simulink model "DISCON_NREL5MW_WaveFF"  (R2022a)
settings: Solver=FixedStepDiscrete  StartTime=0.0  StopTime=inf  FixedStep=Control.TimeStep  RelTol=1e-3
values from neighbouring files (symbols this model uses):
  Gd_Fwave = c2d(Sys{OperatingPoint}('omega_r','F_{hydro}'),Control.TimeStep,'tustin')    [ControlParams_NREL5MW.m]
  Gd_Mwave = c2d(Sys{OperatingPoint}('omega_r','M_{hydro}'),Control.TimeStep,'tustin')    [ControlParams_NREL5MW.m]
  InvGp = inv(Gp)    [ControlParams_NREL5MW.m]
  Kff_gain = 0.3    [InitCompDISCON.m]
undefined symbols (not defined in the file or in its folder): Control
settings Model: Creator=evansolingen  LastModifiedBy=Amr Hegazy
settings SolverCC: AlgebraicLoopSolver=TrustRegion
settings DataIOCC: LimitDataPoints=on  SaveFormat=Array  SignalLoggingSaveFormat=ModelDataLogs  SaveOutput=off  SignalLogging=off  SaveTime=off  ReturnWorkspaceOutputs=off
settings OptimizationCC: ExpressionDepthLimit=2147483647  LifeSpan=inf
settings DebuggingCC: UnderspecifiedInitializationDetection=Classic  MergeDetectMultiDrivingBlocksExec=none  SolverPrmCheckMsg=warning  MultiTaskDSMMsg=warning  MultiTaskCondExecSysMsg=none  FcnCallInpInsideContextMsg=warning  UnconnectedInputMsg=warning  UnconnectedOutputMsg=warning  UnconnectedLineMsg=warning  AllowSymbolicDim=off  StateNameClashWarn=warning  SFUnexpectedBacktrackingDiag=warning  SFNoUnconditionalDefaultTransitionDiag=warning  SFExecutionAtInitializationDiag=none  SFMachineParentedDataDiag=warning  ArithmeticOperatorsInVariantConditions=warning
settings HardwareCC: ProdBitPerPointer=32  ProdBitPerSizeT=32  ProdBitPerPtrDiffT=32  ProdLargestAtomicFloat=None  ProdIntDivRoundTo=Undefined  ProdEndianess=Unspecified  ProdWordSize=32  ProdHWDeviceType=32-bit Generic
settings ModelReferenceCC: UpdateModelReferenceTargets=Force  PropagateSignalLabelsOutOfModel=off
settings SFSimCC: SimUseLocalCustomCode=off  SimParseCustomCode=off  CustomCodeUndefinedFunction=UseInterfaceOnly
settings RTWCC: Description=DISCON DLL Target (for use with GH BLADED)  SystemTargetFile=discon.tlc  TemplateMakefile=discon_vc.tmf  RTWUseLocalCustomCode=off
settings CodeAppCC: StateflowObjectComments=on
settings GRTTargetCC: TargetLangStandard=C89/C90 (ANSI)  CombineOutputUpdateFcns=off  GRTInterface=on  UseToolchainInfoCompliant=off  ExtModeMexFile=noextcomm
settings ConfigComp: CovMetricSettings=dw  CovSaveCumulativeToWorkspaceVar=on  CovSaveSingleToWorkspaceVar=on  CovExternalEMLEnable=off

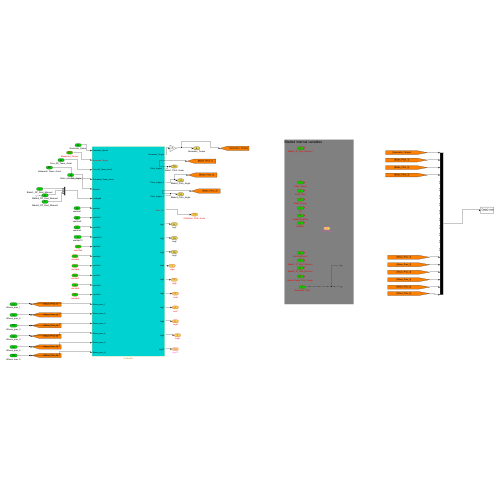
[thumbnail: Simulink's stored preview of the top-level diagram]
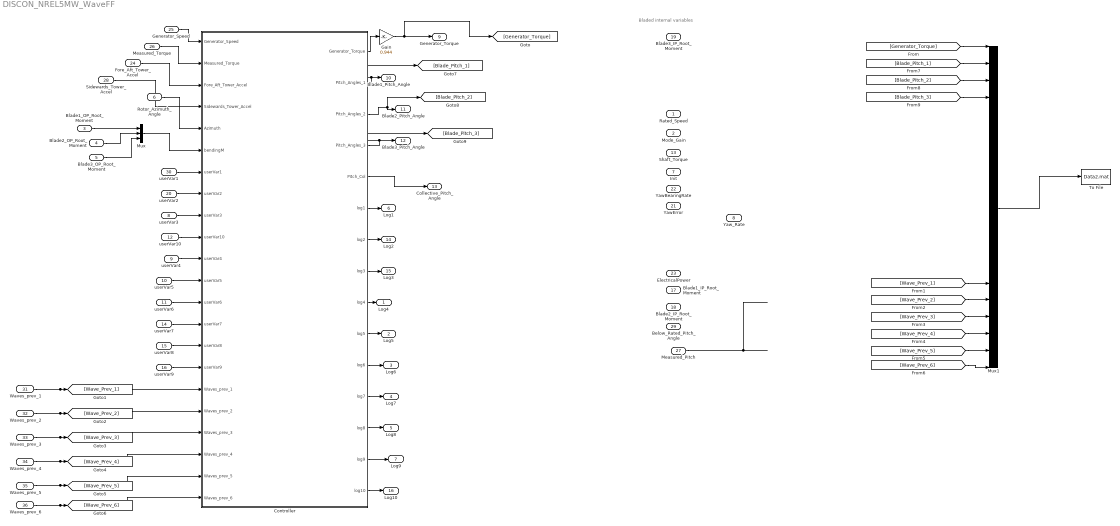
== system DISCON_NREL5MW_WaveFF ==
  note: Bladed internal variables
  Rated_Speed : Inport  PortDimensions=1
  Mode_Gain : Inport  Port=2  PortDimensions=1
  Blade1_OP_Root_Moment : Inport  Port=3  PortDimensions=1
  Blade2_OP_Root_Moment : Inport  Port=4  PortDimensions=1
  Blade3_OP_Root_Moment : Inport  Port=5  PortDimensions=1
  Rotor_Azimuth_Angle : Inport  Port=6  PortDimensions=1
  Init : Inport  Port=7  PortDimensions=1
  userVar3 : Inport  Port=8  PortDimensions=1
  userVar4 : Inport  Port=9  PortDimensions=1
  userVar5 : Inport  Port=10  PortDimensions=1
  userVar6 : Inport  Port=11  PortDimensions=1
  userVar10 : Inport  Port=12  PortDimensions=1
  Shaft_Torque : Inport  Port=13  PortDimensions=1
  userVar7 : Inport  Port=14  PortDimensions=1
  userVar8 : Inport  Port=15  PortDimensions=1
  userVar9 : Inport  Port=16  PortDimensions=1
  Blade1_IP_Root_Moment : Inport  Port=17  PortDimensions=1
  Blade2_IP_Root_Moment : Inport  Port=18  PortDimensions=1
  Blade3_IP_Root_Moment : Inport  Port=19  PortDimensions=1
  userVar2 : Inport  Port=20  PortDimensions=1
  YawError : Inport  Port=21  PortDimensions=1
  YawBearingRate : Inport  Port=22  PortDimensions=1
  ElectricalPower : Inport  Port=23  PortDimensions=1
  Fore_Aft_Tower_Accel : Inport  Port=24  PortDimensions=1
  Generator_Speed : Inport  Port=25  PortDimensions=1
  Measured_Torque : Inport  Port=26  PortDimensions=1
  Measured_Pitch : Inport  Port=27  PortDimensions=1
  Sidewards_Tower_Accel : Inport  Port=28  PortDimensions=1
  Below_Rated_Pitch_Angle : Inport  Port=29  PortDimensions=1
  userVar1 : Inport  Port=30  PortDimensions=1
  Waves_prev_1 : Inport  Port=31  PortDimensions=1
  Waves_prev_2 : Inport  Port=32  PortDimensions=1
  Waves_prev_3 : Inport  Port=33  PortDimensions=1
  Waves_prev_4 : Inport  Port=34  PortDimensions=1
  Waves_prev_5 : Inport  Port=35  PortDimensions=1
  Waves_prev_6 : Inport  Port=36  PortDimensions=1
  Controller : Subsystem
  Gain : Gain  Gain=0.944
  Mux : Mux  Inputs=3
  Mux1 : Mux  Inputs=20
  To File : ToFile  Filename=Data2.mat
  Log4 : Outport  PortDimensions=1  VectorParamsAs1DForOutWhenUnconnected=off
  Log5 : Outport  Port=2  PortDimensions=1  VectorParamsAs1DForOutWhenUnconnected=off
  Log6 : Outport  Port=3  PortDimensions=1  VectorParamsAs1DForOutWhenUnconnected=off
  Log7 : Outport  Port=4  PortDimensions=1  VectorParamsAs1DForOutWhenUnconnected=off
  Log8 : Outport  Port=5  PortDimensions=1  VectorParamsAs1DForOutWhenUnconnected=off
  Log1 : Outport  Port=6  PortDimensions=1  VectorParamsAs1DForOutWhenUnconnected=off
  Log9 : Outport  Port=7  PortDimensions=1  VectorParamsAs1DForOutWhenUnconnected=off
  Yaw_Rate : Outport  Port=8  PortDimensions=1  VectorParamsAs1DForOutWhenUnconnected=off
  Generator_Torque : Outport  Port=9  PortDimensions=1  VectorParamsAs1DForOutWhenUnconnected=off
  Blade1_Pitch_Angle : Outport  Port=10  PortDimensions=1  VectorParamsAs1DForOutWhenUnconnected=off
  Blade2_Pitch_Angle : Outport  Port=11  PortDimensions=1  VectorParamsAs1DForOutWhenUnconnected=off
  Blade3_Pitch_Angle : Outport  Port=12  PortDimensions=1  VectorParamsAs1DForOutWhenUnconnected=off
  Collective_Pitch_Angle : Outport  Port=13  PortDimensions=1  VectorParamsAs1DForOutWhenUnconnected=off
  Log2 : Outport  Port=14  PortDimensions=1  VectorParamsAs1DForOutWhenUnconnected=off
  Log3 : Outport  Port=15  PortDimensions=1  VectorParamsAs1DForOutWhenUnconnected=off
  Log10 : Outport  Port=16  PortDimensions=1  VectorParamsAs1DForOutWhenUnconnected=off
  wires:
  Fore_Aft_Tower_Accel/1 -> Controller/3(Fore_Aft_Tower_Accel)
  Measured_Pitch/1 -> ?
  ? -> ?
  Generator_Speed/1 -> Controller/1(Generator_Speed)
  Controller/1(Generator_Torque) -> Gain/1
  userVar3/1 -> Controller/9(userVar3)
  Gain/1 -> Generator_Torque/1, [Generator_Torque]
  Measured_Torque/1 -> Controller/2(Measured_Torque)
  Sidewards_Tower_Accel/1 -> Controller/4(Sidewards_Tower_Accel)
  Rotor_Azimuth_Angle/1 -> Controller/5(Azimuth)
  Blade1_OP_Root_Moment/1 -> Mux/1
  Blade2_OP_Root_Moment/1 -> Mux/2
  Blade3_OP_Root_Moment/1 -> Mux/3
  Mux/1 -> Controller/6(bendingM)
  Controller/2(Pitch_Angles_1) -> Blade1_Pitch_Angle/1, [Blade_Pitch_1]
  Controller/3(Pitch_Angles_2) -> [Blade_Pitch_2], Blade2_Pitch_Angle/1
  Controller/4(Pitch_Angles_3) -> Blade3_Pitch_Angle/1, [Blade_Pitch_3]
  Controller/5(Pitch_Col) -> Collective_Pitch_Angle/1
  userVar1/1 -> Controller/7(userVar1)
  userVar2/1 -> Controller/8(userVar2)
  userVar10/1 -> Controller/10(userVar10)
  Mux1/1 -> To File/1
  [Generator_Torque] -> Mux1/1
  Waves_prev_1/1 -> Controller/17(Waves_prev_1), [Wave_Prev_1]
  Waves_prev_2/1 -> Controller/18(Waves_prev_2), [Wave_Prev_2]
  Waves_prev_3/1 -> Controller/19(Waves_prev_3), [Wave_Prev_3]
  Waves_prev_4/1 -> Controller/20(Waves_prev_4), [Wave_Prev_4]
  Waves_prev_5/1 -> Controller/21(Waves_prev_5), [Wave_Prev_5]
  Waves_prev_6/1 -> Controller/22(Waves_prev_6), [Wave_Prev_6]
  [Wave_Prev_6] -> Mux1/20
  [Wave_Prev_5] -> Mux1/19
  [Wave_Prev_4] -> Mux1/18
  [Wave_Prev_3] -> Mux1/17
  [Wave_Prev_2] -> Mux1/16
  [Wave_Prev_1] -> Mux1/15
  [Blade_Pitch_1] -> Mux1/2
  [Blade_Pitch_2] -> Mux1/3
  [Blade_Pitch_3] -> Mux1/4
  userVar4/1 -> Controller/11(userVar4)
  userVar5/1 -> Controller/12(userVar5)
  userVar6/1 -> Controller/13(userVar6)
  userVar7/1 -> Controller/14(userVar7)
  userVar8/1 -> Controller/15(userVar8)
  userVar9/1 -> Controller/16(userVar9)
  Controller/6(log1) -> Log1/1
  Controller/7(log2) -> Log2/1
  Controller/8(log3) -> Log3/1
  Controller/10(log5) -> Log5/1
  Controller/12(log7) -> Log7/1
  Controller/13(log8) -> Log8/1
  Controller/9(log4) -> Log4/1
  Controller/15(log10) -> Log10/1
  Controller/11(log6) -> Log6/1
  Controller/14(log9) -> Log9/1

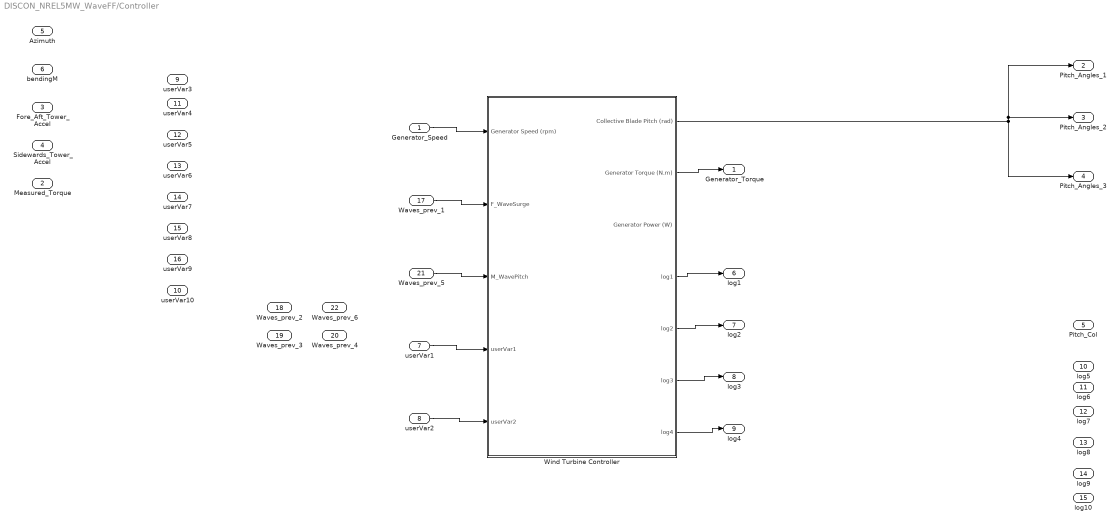
== system DISCON_NREL5MW_WaveFF/Controller ==
  Generator_Speed : Inport
  Measured_Torque : Inport  Port=2
  Fore_Aft_Tower_Accel : Inport  Port=3
  Sidewards_Tower_Accel : Inport  Port=4  PortDimensions=1
  Azimuth : Inport  Port=5  PortDimensions=1
  bendingM : Inport  Port=6
  userVar1 : Inport  Port=7  PortDimensions=1
  userVar2 : Inport  Port=8  PortDimensions=1
  userVar3 : Inport  Port=9  PortDimensions=1
  userVar10 : Inport  Port=10  PortDimensions=1
  userVar4 : Inport  Port=11  PortDimensions=1
  userVar5 : Inport  Port=12  PortDimensions=1
  userVar6 : Inport  Port=13  PortDimensions=1
  userVar7 : Inport  Port=14  PortDimensions=1
  userVar8 : Inport  Port=15  PortDimensions=1
  userVar9 : Inport  Port=16  PortDimensions=1
  Waves_prev_1 : Inport  Port=17  PortDimensions=1
  Waves_prev_2 : Inport  Port=18  PortDimensions=1
  Waves_prev_3 : Inport  Port=19  PortDimensions=1
  Waves_prev_4 : Inport  Port=20  PortDimensions=1
  Waves_prev_5 : Inport  Port=21  PortDimensions=1
  Waves_prev_6 : Inport  Port=22  PortDimensions=1
  Wind Turbine Controller : Subsystem
  Generator_Torque : Outport  VectorParamsAs1DForOutWhenUnconnected=off
  Pitch_Angles_1 : Outport  Port=2  PortDimensions=1  VectorParamsAs1DForOutWhenUnconnected=off
  Pitch_Angles_2 : Outport  Port=3  PortDimensions=1  VectorParamsAs1DForOutWhenUnconnected=off
  Pitch_Angles_3 : Outport  Port=4  PortDimensions=1  VectorParamsAs1DForOutWhenUnconnected=off
  Pitch_Col : Outport  Port=5  PortDimensions=1  VectorParamsAs1DForOutWhenUnconnected=off
  log1 : Outport  Port=6  PortDimensions=1  VectorParamsAs1DForOutWhenUnconnected=off
  log2 : Outport  Port=7  PortDimensions=1  VectorParamsAs1DForOutWhenUnconnected=off
  log3 : Outport  Port=8  PortDimensions=1  VectorParamsAs1DForOutWhenUnconnected=off
  log4 : Outport  Port=9  PortDimensions=1  VectorParamsAs1DForOutWhenUnconnected=off
  log5 : Outport  Port=10  PortDimensions=1  VectorParamsAs1DForOutWhenUnconnected=off
  log6 : Outport  Port=11  PortDimensions=1  VectorParamsAs1DForOutWhenUnconnected=off
  log7 : Outport  Port=12  PortDimensions=1  VectorParamsAs1DForOutWhenUnconnected=off
  log8 : Outport  Port=13  PortDimensions=1  VectorParamsAs1DForOutWhenUnconnected=off
  log9 : Outport  Port=14  PortDimensions=1  VectorParamsAs1DForOutWhenUnconnected=off
  log10 : Outport  Port=15  PortDimensions=1  VectorParamsAs1DForOutWhenUnconnected=off
  wires:
  Wind Turbine Controller/2(Generator Torque (N.m)) -> Generator_Torque/1
  Waves_prev_5/1 -> Wind Turbine Controller/3(M_WavePitch)
  Waves_prev_1/1 -> Wind Turbine Controller/2(F_WaveSurge)
  Generator_Speed/1 -> Wind Turbine Controller/1(Generator Speed (rpm))
  userVar1/1 -> Wind Turbine Controller/4(userVar1)
  userVar2/1 -> Wind Turbine Controller/5(userVar2)
  Wind Turbine Controller/4(log1) -> log1/1
  Wind Turbine Controller/5(log2) -> log2/1
  Wind Turbine Controller/6(log3) -> log3/1
  Wind Turbine Controller/7(log4) -> log4/1
  Wind Turbine Controller/1(" Collective Blade Pitch (rad)") -> Pitch_Angles_2/1, Pitch_Angles_1/1, Pitch_Angles_3/1

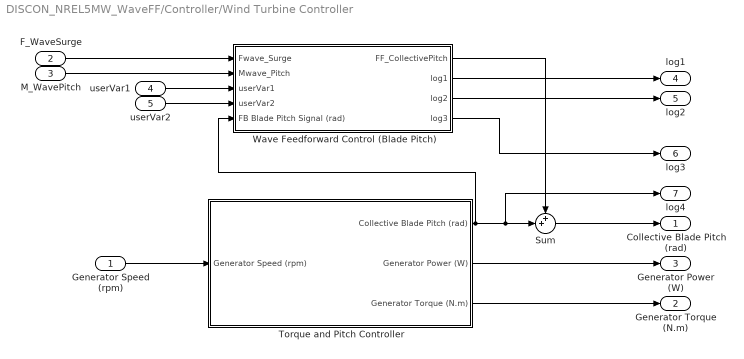
== system DISCON_NREL5MW_WaveFF/Controller/Wind Turbine Controller ==
  Generator Speed (rpm) : Inport
  F_WaveSurge : Inport  Port=2
  M_WavePitch : Inport  Port=3
  userVar1 : Inport  Port=4  PortDimensions=1
  userVar2 : Inport  Port=5  PortDimensions=1
  Sum : Sum  Inputs=++|
  Torque and Pitch Controller : Subsystem
  Wave Feedforward Control (Blade Pitch) : Subsystem
  " Collective Blade Pitch (rad)" : Outport
  Generator Torque (N.m) : Outport  Port=2
  Generator Power (W) : Outport  Port=3
  log1 : Outport  Port=4  PortDimensions=1  VectorParamsAs1DForOutWhenUnconnected=off
  log2 : Outport  Port=5  PortDimensions=1  VectorParamsAs1DForOutWhenUnconnected=off
  log3 : Outport  Port=6  PortDimensions=1  VectorParamsAs1DForOutWhenUnconnected=off
  log4 : Outport  Port=7  PortDimensions=1  VectorParamsAs1DForOutWhenUnconnected=off
  wires:
  Generator Speed (rpm)/1 -> Torque and Pitch Controller/1(Generator Speed (rpm))
  Torque and Pitch Controller/2(Generator Power (W)) -> Generator Power (W)/1
  Torque and Pitch Controller/3(Generator Torque (N.m)) -> Generator Torque (N.m)/1
  Wave Feedforward Control (Blade Pitch)/1(FF_CollectivePitch) -> Sum/1
  Torque and Pitch Controller/1(" Collective Blade Pitch (rad)") -> Wave Feedforward Control (Blade Pitch)/5(FB Blade Pitch Signal (rad)), log4/1, Sum/2
  Sum/1 -> " Collective Blade Pitch (rad)"/1
  Wave Feedforward Control (Blade Pitch)/2(log1) -> log1/1
  Wave Feedforward Control (Blade Pitch)/3(log2) -> log2/1
  Wave Feedforward Control (Blade Pitch)/4(log3) -> log3/1
  userVar1/1 -> Wave Feedforward Control (Blade Pitch)/3(userVar1)
  userVar2/1 -> Wave Feedforward Control (Blade Pitch)/4(userVar2)
  F_WaveSurge/1 -> Wave Feedforward Control (Blade Pitch)/1(Fwave_Surge)
  M_WavePitch/1 -> Wave Feedforward Control (Blade Pitch)/2(Mwave_Pitch)

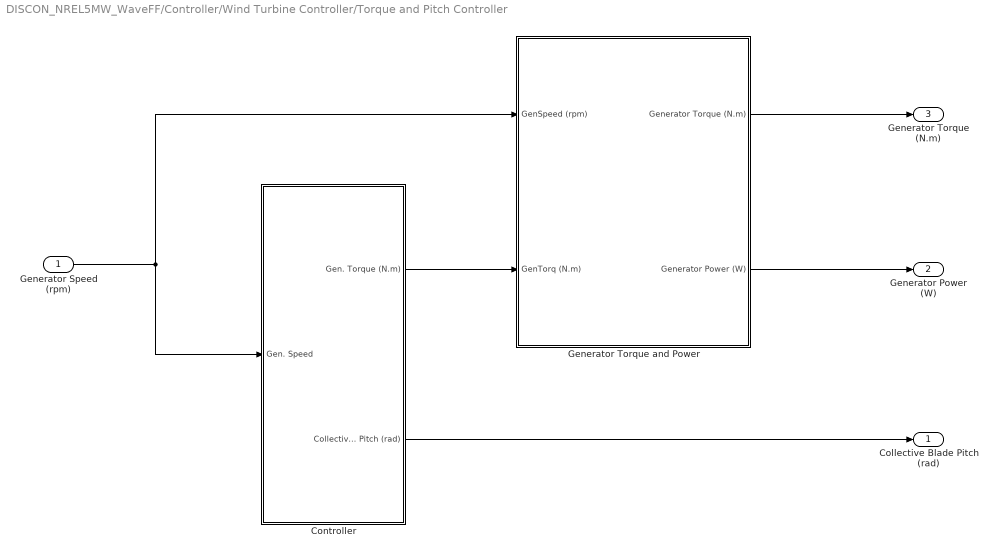
== system DISCON_NREL5MW_WaveFF/Controller/Wind Turbine Controller/Torque and Pitch Controller ==
  Generator Speed (rpm) : Inport
  Controller : Subsystem
  Generator Torque and Power : Subsystem
  " Collective Blade Pitch (rad)" : Outport
  Generator Power (W) : Outport  Port=2
  Generator Torque (N.m) : Outport  Port=3
  wires:
  Controller/1(Gen. Torque (N.m)) -> Generator Torque and Power/2(GenTorq (N.m))
  Generator Torque and Power/1(Generator Torque (N.m)) -> Generator Torque (N.m)/1
  Generator Torque and Power/2(Generator Power (W)) -> Generator Power (W)/1
  Generator Speed (rpm)/1 -> Generator Torque and Power/1(GenSpeed (rpm)), Controller/1(Gen. Speed)
  Controller/2(Collective Blade Pitch (rad)) -> " Collective Blade Pitch (rad)"/1

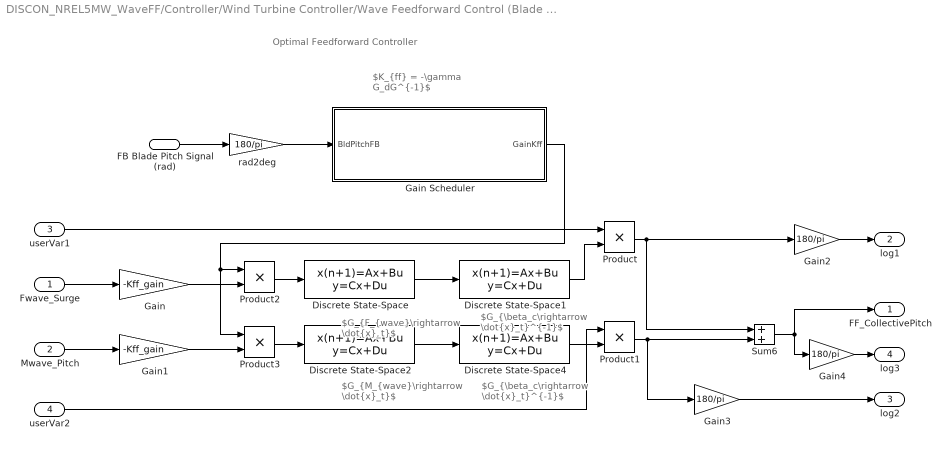
== system DISCON_NREL5MW_WaveFF/Controller/Wind Turbine Controller/Wave Feedforward Control (Blade Pitch) ==
  note: $K_{ff} = -\gamma G_dG^{-1}$
  note: Optimal Feedforward Controller
  note: $G_{F_{wave}\rightarrow \dot{x}_t}$
  note: $G_{M_{wave}\rightarrow \dot{x}_t}$
  note: $G_{\beta_c\rightarrow \dot{x}_t}^{-1}$
  note: $G_{\beta_c\rightarrow \dot{x}_t}^{-1}$
  Fwave_Surge : Inport
  Mwave_Pitch : Inport  Port=2
  userVar1 : Inport  Port=3  PortDimensions=1
  userVar2 : Inport  Port=4  PortDimensions=1
  FB Blade Pitch Signal (rad) : Inport  Port=5
  Discrete State-Space : DiscreteStateSpace  A=Gd_Fwave.A  B=Gd_Fwave.B  C=Gd_Fwave.C  D=Gd_Fwave.D  SampleTime=Control.TimeStep
  Discrete State-Space1 : DiscreteStateSpace  A=InvGp.A  B=InvGp.B  C=InvGp.C  D=InvGp.D  SampleTime=Control.TimeStep
  Discrete State-Space2 : DiscreteStateSpace  A=Gd_Mwave.A  B=Gd_Mwave.B  C=Gd_Mwave.C  D=Gd_Mwave.D  SampleTime=Control.TimeStep
  Discrete State-Space4 : DiscreteStateSpace  A=InvGp.A  B=InvGp.B  C=InvGp.C  D=InvGp.D  SampleTime=Control.TimeStep
  Gain : Gain  Gain=-Kff_gain
  Gain Scheduler : MATLAB Function  TreatAsAtomicUnit=on
  Gain1 : Gain  Gain=-Kff_gain
  Gain2 : Gain  Gain=180/pi
  Gain3 : Gain  Gain=180/pi
  Gain4 : Gain  Gain=180/pi
  Product{,1..3} (4 alike) : Product
  Sum6 : Sum
  rad2deg : Gain  Gain=180/pi
  FF_CollectivePitch : Outport
  log1 : Outport  Port=2  PortDimensions=1  VectorParamsAs1DForOutWhenUnconnected=off
  log2 : Outport  Port=3  PortDimensions=1  VectorParamsAs1DForOutWhenUnconnected=off
  log3 : Outport  Port=4  PortDimensions=1  VectorParamsAs1DForOutWhenUnconnected=off
  wires:
  Fwave_Surge/1 -> Gain/1
  Mwave_Pitch/1 -> Gain1/1
  Sum6/1 -> FF_CollectivePitch/1, Gain4/1
  Discrete State-Space2/1 -> Discrete State-Space4/1
  Discrete State-Space/1 -> Discrete State-Space1/1
  userVar1/1 -> Product/1
  userVar2/1 -> Product1/1
  Gain2/1 -> log1/1
  Gain3/1 -> log2/1
  Gain4/1 -> log3/1
  Discrete State-Space1/1 -> Product/2
  Product/1 -> Sum6/1, Gain2/1
  Gain/1 -> Product2/2
  Discrete State-Space4/1 -> Product1/2
  Product1/1 -> Sum6/2, Gain3/1
  Gain1/1 -> Product3/2
  rad2deg/1 -> Gain Scheduler/1(BldPitchFB)
  FB Blade Pitch Signal (rad)/1 -> rad2deg/1
  Product2/1 -> Discrete State-Space/1
  Gain Scheduler/1(GainKff) -> Product3/1, Product2/1
  Product3/1 -> Discrete State-Space2/1

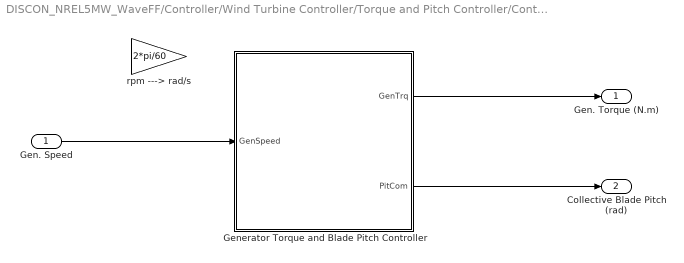
== system DISCON_NREL5MW_WaveFF/Controller/Wind Turbine Controller/Torque and Pitch Controller/Controller ==
  Gen. Speed : Inport
  Generator Torque and Blade Pitch Controller : MATLAB Function  TreatAsAtomicUnit=on
  rpm ---> rad/s : Gain  Gain=2*pi/60
  Gen. Torque (N.m) : Outport
  Collective Blade Pitch (rad) : Outport  Port=2
  wires:
  Gen. Speed/1 -> Generator Torque and Blade Pitch Controller/1(GenSpeed)
  Generator Torque and Blade Pitch Controller/1(GenTrq) -> Gen. Torque (N.m)/1
  Generator Torque and Blade Pitch Controller/2(PitCom) -> Collective Blade Pitch (rad)/1

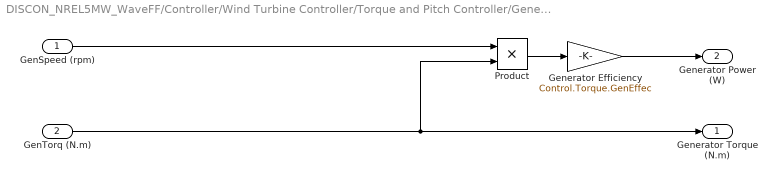
== system DISCON_NREL5MW_WaveFF/Controller/Wind Turbine Controller/Torque and Pitch Controller/Generator Torque and Power ==
  GenSpeed (rpm) : Inport
  GenTorq (N.m) : Inport  Port=2
  Generator Efficiency : Gain  Gain=Control.Torque.GenEffec
  Product : Product
  Generator Torque (N.m) : Outport
  Generator Power (W) : Outport  Port=2
  wires:
  Generator Efficiency/1 -> Generator Power (W)/1
  GenTorq (N.m)/1 -> Generator Torque (N.m)/1, Product/2
  Product/1 -> Generator Efficiency/1
  GenSpeed (rpm)/1 -> Product/1

== matlab function DISCON_NREL5MW_WaveFF/Controller/Wind Turbine Controller/Wave Feedforward Control (Blade Pitch)/Gain Scheduler ==
  data: GainKff output; BldPitchFB input
function GainKff = GainScheduler(BldPitchFB)


% Specifying the operating point based on gain scheduling with respect to
% the feedback blade pitch signal

p1 =   1.378e-06;
p2 =   -0.000122;
p3 =   0.004176;
p4 =    -0.06736;
p5 =      0.4593;
p6 =      0.1538;

GainKff  = p1*BldPitchFB^5 + p2*BldPitchFB^4 + p3*BldPitchFB^3 + p4*BldPitchFB^2 + p5*BldPitchFB + p6;

== matlab function DISCON_NREL5MW_WaveFF/Controller/Wind Turbine Controller/Torque and Pitch Controller/Controller/Generator Torque and Blade Pitch Controller ==
  data: GenTrq output; GenSpeed input; PitCom output; Control parameter
function [GenTrq, PitCom] = Controller(GenSpeed, Control)

%% Definition of the variables used in the script
% LPF_CornerFreq: Corner frequency (-3dB point) in the recursive, single-pole, low-pass filter, rad/s. -- chosen to be 1/4 the blade edgewise natural frequency ( 1/4 of approx. 1Hz = 0.25Hz = 1.570796rad/s)
% TimeStep      : Simulation time step (s)
% PC_DT         : Communication interval for pitch  controller, sec.
% PC_KI         : Integral gain for pitch controller at rated pitch (zero), (-).
% PC_KK         : Pitch angle where the the derivative of the aerodynamic power w.r.t. pitch has increased by a factor of two relative to the derivative at rated pitch (zero), rad.
% PC_KP         : Proportional gain for pitch controller at rated pitch (zero), sec.
% PC_MaxPit     : Maximum pitch setting in pitch controller, rad.
% PC_MaxRat     : Maximum pitch  rate (in absolute value) in pitch  controller, rad/s.
% PC_MinPit     : Minimum pitch setting in pitch controller, rad.
% PC_RefSpd     : Desired (reference) HSS speed for pitch controller, rad/s.
% PitCom        : Commanded pitch of each blade the last time the controller was called, rad.
% PitComI       : Integral term of command pitch, rad.
% PitComP       : Proportional term of command pitch, rad.
% PitComT       : Total command pitch based on the sum of the proportional and integral terms, rad.
% PitRate       : Pitch rates of each blade based on the current pitch angles and current pitch command, rad/s.
% SpdErr        : Current speed error, rad/s.
% TrqRate       : Torque rate based on the current and last torque commands, N-m/s.
% VS_CtInSp     : Transitional generator speed (HSS side) between regions 1 and 1 1/2, rad/s.
% VS_DT         : Communication interval for torque controller, sec.
% VS_MaxRat     : Maximum torque rate (in absolute value) in torque controller, N-m/s.
% VS_MaxTq      : Maximum generator torque in Region 3 (HSS side), N-m. -- chosen to be 10% above VS_RtTq = 43.09355kNm
% VS_Rgn2K      : Generator torque constant in Region 2 (HSS side), N-m/(rad/s)^2.
% VS_Rgn2Sp     : Transitional generator speed (HSS side) between regions 1 1/2 and 2, rad/s.
% VS_Rgn3MP     : Minimum pitch angle at which the torque is computed as if we are in region 3 regardless of the generator speed, rad. -- chosen to be 1.0 degree above PC_MinPit
% VS_RtGnSp     : Rated generator speed (HSS side), rad/s. -- chosen to be 99% of PC_RefSpd
% VS_RtPwr      : Rated generator generator power in Region 3, Watts. -- chosen to be 5MW divided by the electrical generator efficiency of 94.4%
% VS_Slope15    : Torque/speed slope of region 1 1/2 cut-in torque ramp , N-m/(rad/s).
% VS_Slope25    : Torque/speed slope of region 2 1/2 induction generator, N-m/(rad/s).
% VS_SlPc       : Rated generator slip percentage in Region 2 1/2, %.
% VS_SySp       : Synchronous speed of region 2 1/2 induction generator, rad/s.
% VS_TrGnSp     : Transitional generator speed (HSS side) between regions 2 and 2 1/2, rad/s.

% Note, each of the above variables is preceeded by the structure and the
% field where they are defined. That structure is called Control, and is
% composed of 4 field, namely, TimeStep, Filters, Torque and Pitch. 

%% Define the persistent variables in the function
persistent GenSpdFilt PitCommand GK SpdErrInt LastGenTorque 

%% Determine some torque control parameters not specified directly
VS_SySp       = Control.Torque.VS_RtGnSp/( 1.0 +  0.01*Control.Torque.VS_SlPc );                                                                         % Synchronous speed of region 2 1/2 induction generator, rad/s.
VS_Slope15    = (Control.Torque.VS_Rgn2K*Control.Torque.VS_Rgn2Sp*Control.Torque.VS_Rgn2Sp )/( Control.Torque.VS_Rgn2Sp - Control.Torque.VS_CtInSp );   % Torque/speed slope of region 1 1/2 cut-in torque ramp , N-m/(rad/s).
VS_Slope25    = ( Control.Torque.VS_RtPwr/Control.Pitch.PC_RefSpd           )/( Control.Torque.VS_RtGnSp - VS_SySp   );                                  % Torque/speed slope of region 2 1/2 induction generator , N-m/(rad/s).

if ( Control.Torque.VS_Rgn2K == 0.0 )
    VS_TrGnSp = VS_SySp;                                           % TRUE, if the torque in Region 2 is flat, and thus, the denominator in the ELSE condition is zero
else
    VS_TrGnSp = ( VS_Slope25 - sqrt( VS_Slope25*( VS_Slope25 - 4.0*Control.Torque.VS_Rgn2K*VS_SySp ) ) )/( 2.0*Control.Torque.VS_Rgn2K );
end

%% Initialize Saved Variables 
if isempty(GenSpdFilt)
    GenSpdFilt = GenSpeed;                                         % This will ensure that generator speed filter will use the initial value of the generator speed on the first pass                
    PitCommand = Control.Pitch.PC_MinPit;                          % This will ensure that the variable speed controller picks the correct control region and the pitch controller picks the correct gain on the first call
    GK         = 1.0/( 1.0 + PitCommand/Control.Pitch.PC_KK );     % This will ensure that the pitch angle is unchanged if the initial SpdErr is zero
    SpdErrInt  = PitCommand/( GK*Control.Pitch.PC_KI );            % This will ensure that the pitch angle is unchanged if the initial SpdErr is zero    
end

%% ============================= Filtering ============================= %%
% Filter the HSS (generator) speed measurement
% NOTE: This is a very simple recursive, single-pole, low-pass filter with exponential smoothing.
Alpha         = exp( -Control.TimeStep * Control.Filters.LPF_CornerFreq );

% Apply the Filter
GenSpeedF = ( 1.0 - Alpha )*GenSpeed + Alpha * GenSpdFilt;

% Update the persistent variable GenSpdFilt (This is to store the value of the presistent variable to be e used in the next time step)
GenSpdFilt = GenSpeedF;
     
%% =================== Variable-Speed Torque Control =================== %%
% Compute the generator torque, which depends on which region we are in:
if(GenSpeedF >= Control.Torque.VS_RtGnSp)||( PitCommand>= Control.Torque.VS_Rgn3MP )                   % We are in region 3 - power is constant
    GenTrq = Control.Torque.VS_RtPwr/Control.Pitch.PC_RefSpd;
elseif(GenSpeedF <= Control.Torque.VS_CtInSp)                                                          % We are in region 1 - torque is zero
    GenTrq = 0.0;
elseif(GenSpeedF <  Control.Torque.VS_Rgn2Sp)                                                          % We are in region 1 1/2 - linear ramp in torque from zero to optimal
    GenTrq = VS_Slope15*( GenSpeedF - Control.Torque.VS_CtInSp );
elseif(GenSpeedF <  VS_TrGnSp)                                                                         % We are in region 2 - optimal torque is proportional to the square of the generator speed
    GenTrq = Control.Torque.VS_Rgn2K*GenSpeedF*GenSpeedF;
else                                                                                                   % We are in region 2 1/2 - simple induction generator transition region
    GenTrq = VS_Slope25*( GenSpeedF - VS_SySp   );
end

% Saturate the commanded torque using the maximum torque limit:
GenTrq  = min( GenTrq, Control.Torque.VS_MaxTq  );                                                     % Saturate the command using the maximum torque limit

% Saturate the commanded torque using the torque rate limit:
if isempty(LastGenTorque)
    LastGenTorque = GenTrq;                                                                            % Initialize the value of LastGenTrq on the first pass only
end

TrqRate = ( GenTrq - LastGenTorque )/Control.TimeStep;                                                 % Torque rate (unsaturated)         
TrqRate = min( max( TrqRate, -Control.Torque.VS_MaxRat ), Control.Torque.VS_MaxRat );                  % Saturate the torque rate using its maximum absolute value
GenTrq  = LastGenTorque + TrqRate*Control.TimeStep;                                                    % Saturate the command using the torque rate limit

% Store the value of LastGenTorque for the next time step:
LastGenTorque = GenTrq;


%% =========================== Pitch Control =========================== %%

% Compute the gain scheduling correction factor based on the previously commanded pitch angle for blade 1:
GK = 1.0/( 1.0 + PitCommand/Control.Pitch.PC_KK );                    

% Compute the current speed error and its integral w.r.t. time;
% saturate the integral term using the pitch angle limits:
SpdErr    = GenSpdFilt - Control.Pitch.PC_RefSpd;                                                     % Current speed error        
IntSpdErr = SpdErrInt + SpdErr*Control.TimeStep;                                                      % Current integral of speed error w.r.t. time             
IntSpdErr = min( max( IntSpdErr, Control.Pitch.PC_MinPit/( GK*Control.Pitch.PC_KI ) ), Control.Pitch. PC_MaxPit/( GK*Control.Pitch.PC_KI ));    % Saturate the integral term using the pitch angle limits, converted to integral speed error limits

% Compute the pitch commands associated with the proportional and integral gains:
PitComP   = GK*Control.Pitch.PC_KP*SpdErr;                                                            % Proportional term          
PitComI   = GK*Control.Pitch.PC_KI*IntSpdErr;                                                         % Integral term (saturated) 

% Superimpose the individual commands to get the total pitch command;
%  saturate the overall command using the pitch angle limits:
PitComT   = PitComP + PitComI;                                                                        % Overall command (unsaturated)       
PitComT   = min( max( PitComT, Control.Pitch.PC_MinPit ), Control.Pitch.PC_MaxPit );                  % Saturate the overall command using the pitch angle limits

% Saturate the overall commanded pitch using the pitch rate limit:
% NOTE: Since the current pitch angle may be different for each blade
% (depending on the type of actuator implemented in the structural
% dynamics model), this pitch rate limit calculation and the 
% resulting overall pitch angle command may be different for each blade.
PitRate   = ( PitComT - PitCommand)/Control.TimeStep;                                                 % Pitch rate of the blades (unsaturated)           
PitRate   = min( max( PitRate, -Control.Pitch.PC_MaxRat ), Control.Pitch.PC_MaxRat );                 % Saturate the pitch rate of the blade using its maximum absolute value

PitCom    = PitCommand + PitRate*Control.TimeStep;                                                    % Saturate the overall command of the blade using the pitch rate limit           
PitCom    = min( max( PitCom, Control.Pitch.PC_MinPit ), Control.Pitch.PC_MaxPit );                   % Saturate the overall command using the pitch angle limits

% Store the persistent variables to be used in the next time step)
PitCommand = PitCom;
SpdErrInt = IntSpdErr;
